simulink model "FIR_FILTER_direct_form"  (R2020b)
settings: Solver=FixedStepAuto  StartTime=0.0  StopTime=10.0  FixedStep=1  RelTol=1e-3
PreLoadFcn:
  | Preload_values
values from neighbouring files (symbols this model uses):
  b0 = 1    [Preload_values.m]
  b1 = 2    [Preload_values.m]
  b2 = 3    [Preload_values.m]
  b3 = 4    [Preload_values.m]
  b4 = 5    [Preload_values.m]
settings Model: Creator=hp  LastModifiedBy=hp
settings DataIOCC: SaveOutput=off  SaveTime=off

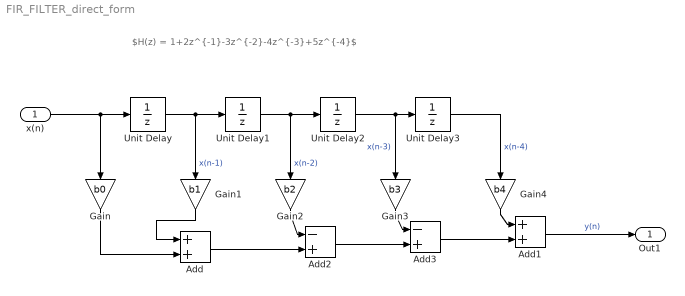
== system FIR_FILTER_direct_form ==
  note: $H(z) = 1+2z^{-1}-3z^{-2}-4z^{-3}+5z^{-4}$
  x(n) : Inport  OutDataTypeStr=double  PortDimensions=1  SampleTime=[1,0]
  Add : Sum
  Add1 : Sum
  Add2 : Sum  Inputs=-+
  Add3 : Sum  Inputs=-+
  Gain : Gain  Gain=b0
  Gain1 : Gain  Gain=b1
  Gain2 : Gain  Gain=b2
  Gain3 : Gain  Gain=b3
  Gain4 : Gain  Gain=b4
  Unit Delay{,1..3} (4 alike) : UnitDelay  SampleTime=-1  HasFrameUpgradeWarning=on
  Out1 : Outport  OutDataTypeStr=double  PortDimensions=1  SampleTime=[1,0]
  wires:
  Unit Delay1/1 -> Unit Delay2/1, Gain2/1  "x(n-2)"
  Add/1 -> Add2/2
  Unit Delay2/1 -> Gain3/1, Unit Delay3/1  "x(n-3)"
  Add3/1 -> Add1/2
  Gain3/1 -> Add3/1
  Gain2/1 -> Add2/1
  Gain1/1 -> Add/1
  Gain/1 -> Add/2
  x(n)/1 -> Unit Delay/1, Gain/1
  Unit Delay3/1 -> Gain4/1  "x(n-4)"
  Unit Delay/1 -> Unit Delay1/1, Gain1/1  "x(n-1)"
  Add2/1 -> Add3/2
  Gain4/1 -> Add1/1
  Add1/1 -> Out1/1  "y(n)"
